simulink model "QCM_2020"  (R2020b)
settings: Solver=FixedStepAuto  StartTime=0.0  StopTime=20  FixedStep=0.01  RelTol=1e-3
undefined symbols (not defined in the file or in its folder): par
settings Model: Creator=maart  LastModifiedBy=Tjeu
settings SolverCC: ZeroCrossAlgorithm=Adaptive
settings DebuggingCC: IgnoredZcDiagnostic=none

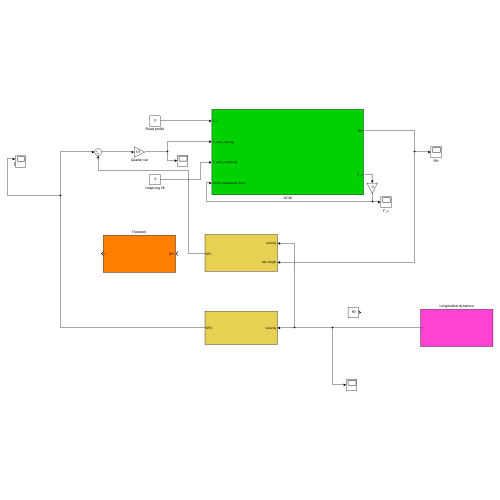
[thumbnail: Simulink's stored preview of the top-level diagram]
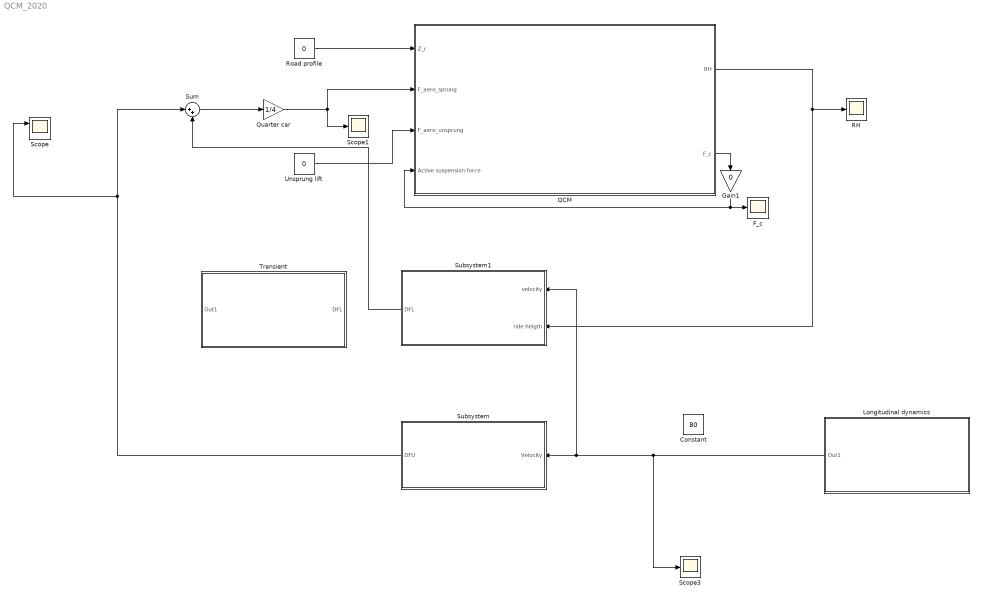
== system QCM_2020 ==
  Constant : Constant  Value=80
  F_c : Scope
  Gain1 : Gain  Gain=0
  Longitudinal dynamics : Subsystem
  QCM : Subsystem
  Quarter car : Gain  Gain=1/4
  RH : Scope
  Road profile : Constant  Value=0
  Scope : Scope  NumInputPorts=2
  Scope1 : Scope
  Scope3 : Scope
  Subsystem : Subsystem
  Subsystem1 : Subsystem
  Sum : Sum  Inputs=|++
  "Transient " : Subsystem
  Unsprung lift : Constant  Value=0
  wires:
  Road profile/1 -> QCM/1(Z_r)
  Unsprung lift/1 -> QCM/3(F_aero_unsprung)
  Sum/1 -> Quarter car/1
  QCM/1(RH) -> Subsystem1/2(ride heigth), RH/1
  Longitudinal dynamics/1(Out1) -> Scope3/1, Subsystem1/1(velocity), Subsystem/1(Velocity)
  Quarter car/1 -> Scope1/1, QCM/2(F_aero_sprung)
  Subsystem/1(DFU) -> Scope/1, Sum/1
  QCM/2(F_c) -> Gain1/1
  Gain1/1 -> QCM/4(Active suspension force), F_c/1
  Subsystem1/1(DFL) -> Sum/2

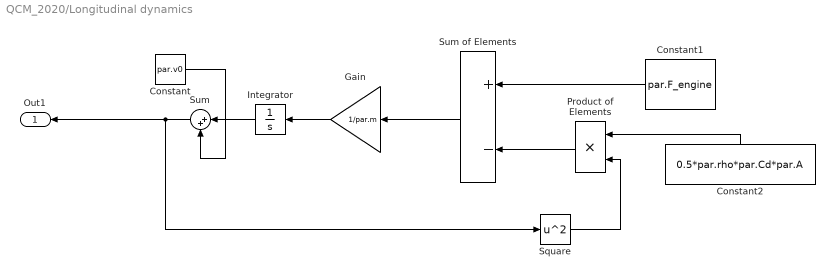
== system QCM_2020/Longitudinal dynamics ==
  Constant : Constant  Value=par.v0
  Constant1 : Constant  Value=par.F_engine
  Constant2 : Constant  Value=0.5*par.rho*par.Cd*par.A
  Gain : Gain  Gain=1/par.m
  Integrator : Integrator
  Product of Elements : Product  Inputs=**
  Square : Math  Operator=square  SaturateOnIntegerOverflow=on
  Sum : Sum  Inputs=|++
  Sum of Elements : Sum  Inputs=+-
  Out1 : Outport
  wires:
  Constant1/1 -> Sum of Elements/1
  Sum of Elements/1 -> Gain/1
  Gain/1 -> Integrator/1
  Product of Elements/1 -> Sum of Elements/2
  Integrator/1 -> Sum/1
  Constant/1 -> Sum/2
  Sum/1 -> Square/1, Out1/1
  Constant2/1 -> Product of Elements/1
  Square/1 -> Product of Elements/2

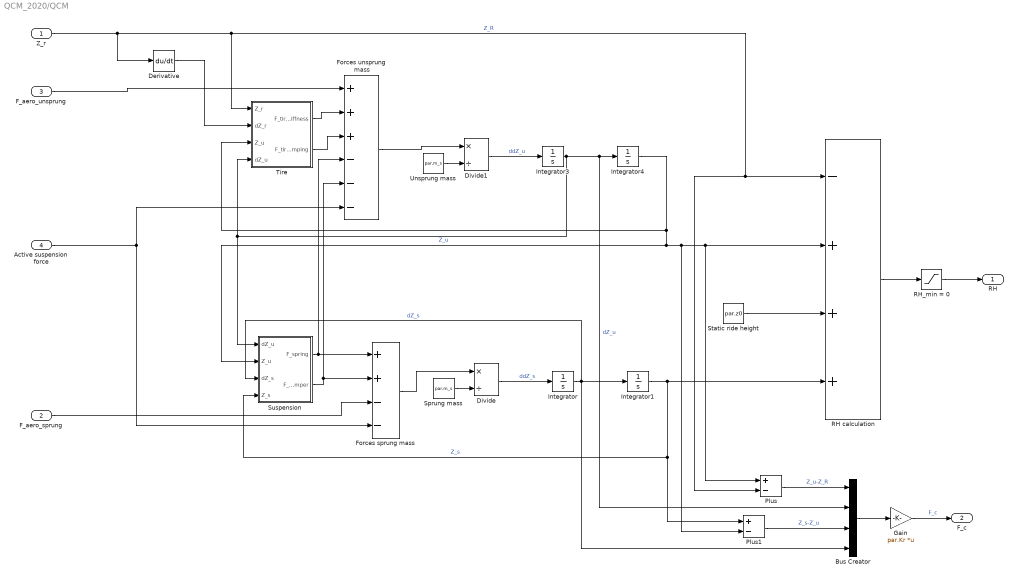
== system QCM_2020/QCM ==
  Z_r : Inport
  F_aero_sprung : Inport  Port=2
  F_aero_unsprung : Inport  Port=3
  Active suspension force : Inport  Port=4
  Bus Creator : BusCreator  Inputs=4
  Derivative : Derivative
  Divide : Product  Inputs=*/
  Divide1 : Product  Inputs=*/
  Forces sprung mass : Sum  Inputs=++--
  Forces unsprung mass : Sum  Inputs=+++---
  Gain : Gain  Gain=par.Kr  Multiplication=Matrix(K*u)
  Integrator{,1,3..4} (4 alike) : Integrator
  Plus : Sum  Inputs=+-
  Plus1 : Sum  Inputs=+-
  RH calculation : Sum  Inputs=-+++
  RH_min = 0 : Saturate  UpperLimit=inf  LowerLimit=0
  Sprung mass : Constant  Value=par.m_s
  Static ride height : Constant  Value=par.z0
  Suspension : Subsystem
  Tire : Subsystem
  Unsprung mass : Constant  Value=par.m_s
  RH : Outport
  F_c : Outport  Port=2
  wires:
  Forces sprung mass/1 -> Divide/1
  Sprung mass/1 -> Divide/2
  Divide/1 -> Integrator/1  "ddZ_s"
  Integrator/1 -> Bus Creator/4, Suspension/3(dZ_s), Integrator1/1  "dZ_s"
  Integrator1/1 -> Plus1/1, Suspension/4(Z_s), RH calculation/4  "Z_s"
  F_aero_sprung/1 -> Forces sprung mass/3
  Integrator3/1 -> Bus Creator/2, Integrator4/1, Tire/4(dZ_u), Suspension/1(dZ_u)  "dZ_u"
  Integrator4/1 -> Tire/3(Z_u), Plus1/2, Plus/1, RH calculation/2, Suspension/2(Z_u)  "Z_u"
  Unsprung mass/1 -> Divide1/2
  Divide1/1 -> Integrator3/1  "ddZ_u"
  Forces unsprung mass/1 -> Divide1/1
  Static ride height/1 -> RH calculation/3
  Z_r/1 -> Derivative/1, Tire/1(Z_r), RH calculation/1, Plus/2  "Z_R"
  Suspension/1(F_spring) -> Forces unsprung mass/4, Forces sprung mass/1
  Suspension/2(F_damper) -> Forces unsprung mass/5, Forces sprung mass/2
  Tire/2(F_tire_damping) -> Forces unsprung mass/3
  Tire/1(F_tire_stiffness) -> Forces unsprung mass/2
  F_aero_unsprung/1 -> Forces unsprung mass/1
  Derivative/1 -> Tire/2(dZ_r)
  RH calculation/1 -> RH_min = 0/1
  RH_min = 0/1 -> RH/1
  Active suspension force/1 -> Forces sprung mass/4, Forces unsprung mass/6
  Plus/1 -> Bus Creator/1  "Z_u-Z_R"
  Plus1/1 -> Bus Creator/3  "Z_s-Z_u"
  Bus Creator/1 -> Gain/1
  Gain/1 -> F_c/1  "F_c"

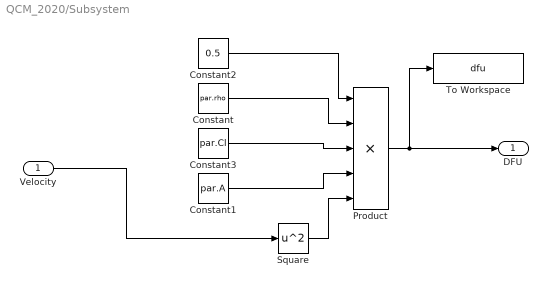
== system QCM_2020/Subsystem ==
  Velocity : Inport
  Constant : Constant  Value=par.rho
  Constant1 : Constant  Value=par.A
  Constant2 : Constant  Value=0.5
  Constant3 : Constant  Value=par.Cl
  Product : Product  Inputs=5
  Square : Math  Operator=square  SaturateOnIntegerOverflow=on
  To Workspace : ToWorkspace  VariableName=dfu  SaveFormat=Timeseries  SampleTime=-1
  DFU : Outport
  wires:
  Constant2/1 -> Product/1
  Constant/1 -> Product/2
  Constant1/1 -> Product/4
  Constant3/1 -> Product/3
  Square/1 -> Product/5
  Product/1 -> DFU/1, To Workspace/1
  Velocity/1 -> Square/1

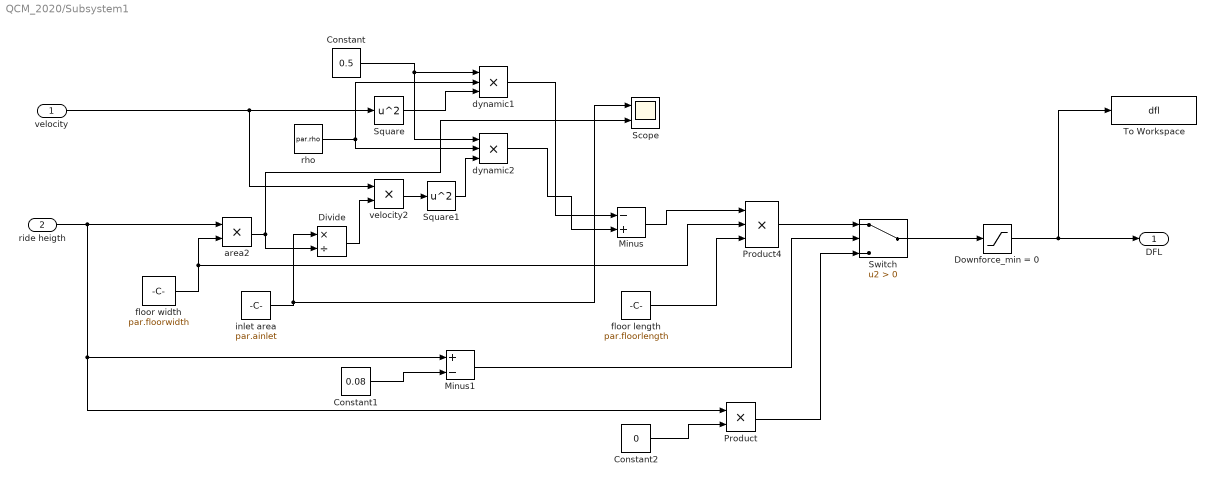
== system QCM_2020/Subsystem1 ==
  velocity : Inport
  ride heigth : Inport  Port=2
  Constant : Constant  Value=0.5
  Constant1 : Constant  Value=0.08
  Constant2 : Constant  Value=0
  Divide : Product  Inputs=*/
  Downforce_min = 0 : Saturate  UpperLimit=Inf  LowerLimit=0
  Minus : Sum  Inputs=-+
  Minus1 : Sum  Inputs=+-
  Product : Product
  Product4 : Product  Inputs=3
  Scope : Scope  NumInputPorts=2
  Square : Math  Operator=square  SaturateOnIntegerOverflow=on
  Square1 : Math  Operator=square  SaturateOnIntegerOverflow=on
  Switch : Switch  Criteria=u2 > Threshold
  To Workspace : ToWorkspace  VariableName=dfl  SaveFormat=Timeseries  SampleTime=-1
  area2 : Product
  dynamic1 : Product  Inputs=3
  dynamic2 : Product  Inputs=3
  floor length : Constant  Value=par.floorlength
  floor width : Constant  Value=par.floorwidth
  inlet area : Constant  Value=par.ainlet
  rho : Constant  Value=par.rho
  velocity2 : Product
  DFL : Outport
  wires:
  Square1/1 -> dynamic2/3
  dynamic1/1 -> Minus/1
  Divide/1 -> velocity2/2
  area2/1 -> Scope/2, Divide/2
  rho/1 -> dynamic1/2, dynamic2/2
  floor width/1 -> Product4/2, area2/2
  velocity/1 -> Square/1, velocity2/1
  dynamic2/1 -> Minus/2
  floor length/1 -> Product4/3
  Minus/1 -> Product4/1
  Square/1 -> dynamic1/3
  Constant/1 -> dynamic2/1, dynamic1/1
  ride heigth/1 -> Product/1, Minus1/1, area2/1
  velocity2/1 -> Square1/1
  inlet area/1 -> Scope/1, Divide/1
  Constant1/1 -> Minus1/2
  Minus1/1 -> Switch/2
  Constant2/1 -> Product/2
  Product/1 -> Switch/3
  Downforce_min = 0/1 -> To Workspace/1, DFL/1
  Product4/1 -> Switch/1
  Switch/1 -> Downforce_min = 0/1

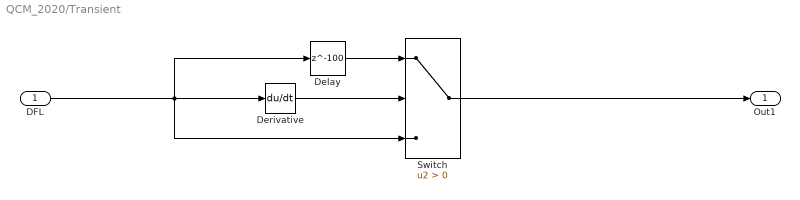
== system QCM_2020/Transient  ==
  DFL : Inport
  Delay : Delay  DelayLength=100
  Derivative : Derivative
  Switch : Switch  Criteria=u2 > Threshold
  Out1 : Outport
  wires:
  DFL/1 -> Switch/3, Delay/1, Derivative/1
  Derivative/1 -> Switch/2
  Delay/1 -> Switch/1
  Switch/1 -> Out1/1

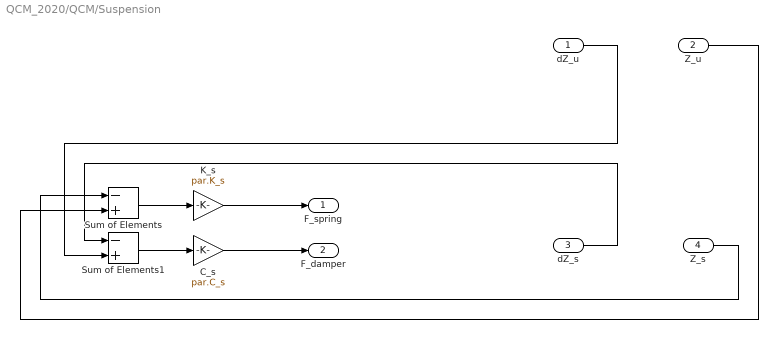
== system QCM_2020/QCM/Suspension ==
  dZ_u : Inport
  Z_u : Inport  Port=2
  dZ_s : Inport  Port=3
  Z_s : Inport  Port=4
  C_s : Gain  Gain=par.C_s
  K_s : Gain  Gain=par.K_s
  Sum of Elements : Sum  Inputs=-+
  Sum of Elements1 : Sum  Inputs=-+
  F_spring : Outport
  F_damper : Outport  Port=2
  wires:
  Z_s/1 -> Sum of Elements/1
  Sum of Elements/1 -> K_s/1
  Sum of Elements1/1 -> C_s/1
  K_s/1 -> F_spring/1
  dZ_u/1 -> Sum of Elements1/2
  Z_u/1 -> Sum of Elements/2
  C_s/1 -> F_damper/1
  dZ_s/1 -> Sum of Elements1/1

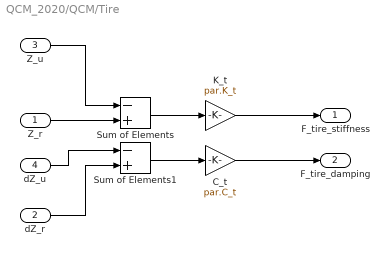
== system QCM_2020/QCM/Tire ==
  Z_r : Inport
  dZ_r : Inport  Port=2
  Z_u : Inport  Port=3
  dZ_u : Inport  Port=4
  C_t : Gain  Gain=par.C_t
  K_t : Gain  Gain=par.K_t
  Sum of Elements : Sum  Inputs=-+
  Sum of Elements1 : Sum  Inputs=-+
  F_tire_stiffness : Outport
  F_tire_damping : Outport  Port=2
  wires:
  Sum of Elements/1 -> K_t/1
  Sum of Elements1/1 -> C_t/1
  K_t/1 -> F_tire_stiffness/1
  C_t/1 -> F_tire_damping/1
  Z_u/1 -> Sum of Elements/1
  Z_r/1 -> Sum of Elements/2
  dZ_u/1 -> Sum of Elements1/1
  dZ_r/1 -> Sum of Elements1/2
